simulink model "AWident"  (Simulink 6.3)
settings: Solver=ode45  StartTime=0.0  StopTime=tend  MaxStep=0.01  RelTol=1e-3
values from neighbouring files (symbols this model uses):
  sigma2v = 0    [zad_2_1.m]    (also in zad_3_1.m = 0.001)
  Tp = 1    [zad_2_1.m]    (also in zad_3_1.m = 0.5)
libraries: simulink x1
settings Model: LastModifiedBy=Maciej

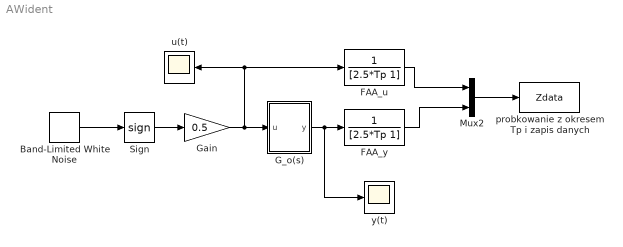
== system AWident ==
  Band-Limited White Noise : simulink/Sources/Band-Limited White Noise  Cov=[0.5]*Tp  Ts=Tp  seed=[23341]
  FAA_u : TransferFcn  Denominator=[2.5*Tp 1]
  FAA_y : TransferFcn  Denominator=[2.5*Tp 1]
  G_o(s) : Subsystem
  Gain : Gain  Gain=0.5
  Mux2 : Mux  Inputs=2
  Sign : Signum  ZeroCross=off
  probkowanie z okresem Tp i zapis danych : ToWorkspace  VariableName=Zdata  SampleTime=Tp  SaveFormat=Array
  u(t) : Scope
  y(t) : Scope
  wires:
  Band-Limited White Noise/1 -> Sign/1
  Sign/1 -> Gain/1
  Gain/1 -> G_o(s)/1(u), FAA_u/1, u(t)/1
  G_o(s)/1(y) -> FAA_y/1, y(t)/1
  FAA_u/1 -> Mux2/1
  FAA_y/1 -> Mux2/2
  Mux2/1 -> probkowanie z okresem Tp i zapis danych/1

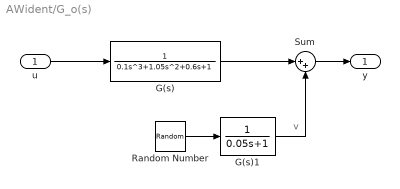
== system AWident/G_o(s) ==
  note: v
  u : Inport
  G(s) : TransferFcn  Denominator=[0.1 1.05 0.6 1]
  G(s)1 : TransferFcn  Denominator=[0.05 1]
  Random Number : RandomNumber  Variance=sigma2v  Seed=159  SampleTime=Tp*0.1
  Sum : Sum  Inputs=|++
  y : Outport
  wires:
  G(s)/1 -> Sum/1
  u/1 -> G(s)/1
  Sum/1 -> y/1
  G(s)1/1 -> Sum/2
  Random Number/1 -> G(s)1/1
